simulink model "Q3"  (R2018b)
settings: Solver=VariableStepAuto  StartTime=0.0  StopTime=50  RelTol=1e-3
values from neighbouring files (symbols this model uses):
  A = double(A2)    [questao3.m]
  B = double(B2)    [questao3.m]
  C2 = [0 1]    [questao3.m]
  D = 0    [questao3.m]
  k = kt(1:length(sys.A))    [questao1.m]    (also in questao3.m = kt(1:length(A)))
  ka = -kt(end)    [questao1.m]    (also in questao3.m)
libraries: simulink x1
settings Model: Creator=bernardo  LastModifiedBy=bernardo

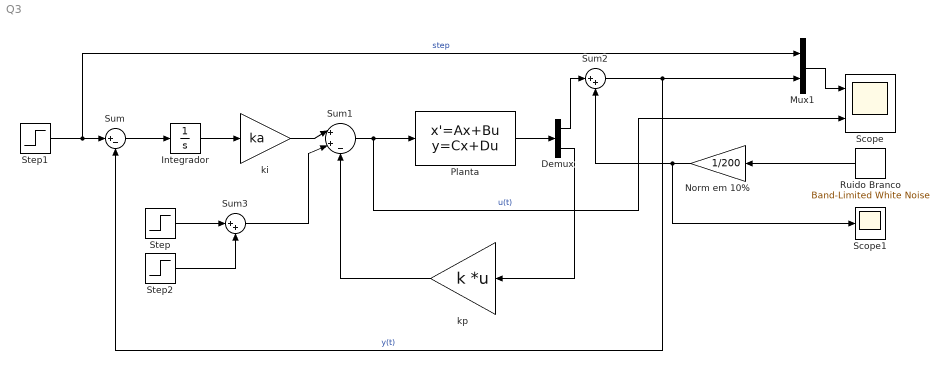
== system Q3 ==
  Demux : Demux  Outputs=[1;length(A)]
  Integrador : Integrator
  Mux1 : Mux  Inputs=2
  Norm em 10% : Gain  Gain=1/200
  Planta : StateSpace  A=A  B=B  C=[C2; eye(length(A))]  D=[D; zeros(length(A),1)]  InitialCondition=0
  Ruido Branco : simulink/Sources/Band-Limited White Noise  Cov=[0.1]  Ts=0.01  seed=[23341]
  Scope : Scope  NumInputPorts=2
  Scope1 : Scope
  Step : Step  Time=20  After=-1/5  SampleTime=0
  Step1 : Step  Time=10  SampleTime=0.01
  Step2 : Step  Time=30  After=1/5  SampleTime=0
  Sum : Sum  Inputs=|+-
  Sum1 : Sum  Inputs=|++-
  Sum2 : Sum  Inputs=|++
  Sum3 : Sum  Inputs=|++
  ki : Gain  Gain=ka
  kp : Gain  Gain=k  Multiplication=Matrix(K*u)
  wires:
  Sum1/1 -> Scope/2, Planta/1  "u(t)"
  kp/1 -> Sum1/3
  Planta/1 -> Demux/1
  Integrador/1 -> ki/1
  ki/1 -> Sum1/1
  Sum/1 -> Integrador/1
  Step1/1 -> Mux1/1, Sum/1  "step"
  Demux/2 -> kp/1
  Ruido Branco/1 -> Norm em 10%/1
  Sum2/1 -> Sum/2, Mux1/2  "y(t)"
  Norm em 10%/1 -> Scope1/1, Sum2/2
  Mux1/1 -> Scope/1
  Step2/1 -> Sum3/2
  Step/1 -> Sum3/1
  Sum3/1 -> Sum1/2
  Demux/1 -> Sum2/1
